simulink model "DAB_IBDC_CONST"  (R2019b)
settings: Solver=ode23t  StartTime=0.0  StopTime=10.0  RelTol=1e-3
libraries: powerlib x18
settings Model: Creator=khduh  LastModifiedBy=khduh

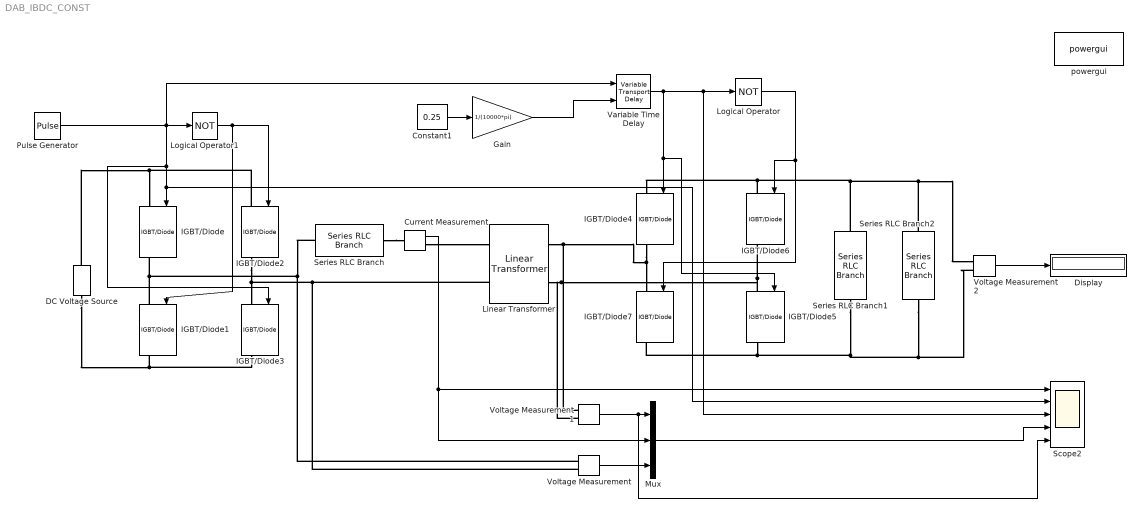
== system DAB_IBDC_CONST ==
  Constant1 : Constant  Value=0.25
  Current Measurement : powerlib/Measurements/Current Measurement  PhasorSimulation=off  OutputType=Complex  PSBequivalent=0
      settings: SourceProductName=Simscape Electrical
  DC Voltage Source : powerlib/Electrical Sources/DC Voltage Source  Amplitude=1000  Measurements=None
      settings: SourceProductName=Simscape Electrical
  Display : Display
  Gain : Gain  Gain=1/(10000*pi)
  IGBT/Diode{,1..7} (8 alike) : powerlib/Power Electronics/IGBT//Diode  Ron=1e-3  Rs=1e5  Cs=inf  Measurements=on
      settings: SourceProductName=Simscape Electrical
  Linear Transformer : powerlib/Elements/Linear Transformer  UNITS=SI  NominalPower=[ 250e6 10000*pi ]  winding1=[500 0 0]  winding2=[250 0 0]  ThreeWindings=off  winding3=[3.15e+05 0.7938 0.084225]  RmLm=[1.0805e+06 2866]  Measurements=None  DataType=on
      settings: SourceProductName=Simscape Electrical
  Logical Operator : Logic  Operator=NOT  AllPortsSameDT=off  OutDataTypeStr=boolean
  Logical Operator1 : Logic  Operator=NOT  AllPortsSameDT=off  OutDataTypeStr=boolean
  Mux : Mux  Inputs=3
  Pulse Generator : DiscretePulseGenerator  PulseType=Time based  Period=1/(10000*pi)  PulseWidth=50
  Scope2 : Scope  NumInputPorts=5
  Series RLC Branch : powerlib/Elements/Series RLC Branch  LConnTagsString=__new0  RConnTagsString=__new0  BranchType=L  Resistance=1  Inductance=.0102e-3  SetiL0=off  InitialCurrent=0  Capacitance=1e-6  Setx0=off  InitialVoltage=0  Measurements=None
      settings: SourceProductName=Simscape Electrical
  Series RLC Branch1 : powerlib/Elements/Series RLC Branch  LConnTagsString=__new0  RConnTagsString=__new0  BranchType=C  Resistance=1  Inductance=.0102e-3  SetiL0=off  InitialCurrent=0  Capacitance=660e-6  Setx0=off  InitialVoltage=0  Measurements=None
      settings: SourceProductName=Simscape Electrical
  Series RLC Branch2 : powerlib/Elements/Series RLC Branch  LConnTagsString=__new0  RConnTagsString=__new0  BranchType=R  Resistance=1  Inductance=.0102e-3  SetiL0=off  InitialCurrent=0  Capacitance=1e-6  Setx0=off  InitialVoltage=0  Measurements=None
      settings: SourceProductName=Simscape Electrical
  Variable Time Delay : VariableTransportDelay  MaximumDelay=10
  Voltage Measurement : powerlib/Measurements/Voltage Measurement  PhasorSimulation=off  OutputType=Complex  PSBequivalent=0
      settings: SourceProductName=Simscape Electrical
  Voltage Measurement1 : powerlib/Measurements/Voltage Measurement  PhasorSimulation=off  OutputType=Complex  PSBequivalent=0
      settings: SourceProductName=Simscape Electrical
  Voltage Measurement2 : powerlib/Measurements/Voltage Measurement  PhasorSimulation=off  OutputType=Complex  PSBequivalent=0
      settings: SourceProductName=Simscape Electrical
  powergui : powerlib/powergui  Priority=1  SimulationMode=Discrete  SampleTime=1e-7  frequency=60  Iterations=50  frequencyindice=0  Pbase=100e6  ErrMax=1e-4  UnitsV=kV  UnitsW=MW  buscounter=0  FunctionMessages=off  echomessages=off  EnableUseOfTLC=off  CurrentSourceSwitches=off  DisableSnubberDevices=off  DisableRonSwitches=off  DisableVfSwitches=off  DisplayEquations=off  AutomaticDiscreteSolvers=off  SolverType=Tustin/Backward Euler (TBE)  Interpol=off  ExternalGateDelay=off  methode=off  Ts=100  x0status=blocks  SPID=on  SwTol=0  HookPort=off  NonlinearTolerance=1e-4  nMaxIteration=100  ContinueOnMaxIteration=off  RestoreLinks=warning  ResistiveCurrentMeasurement=off  Frange=[0:2:500]  Ylog=off  Xlog=on  ShowGrid=off  save=off  variable=ZData  structure=0  ZoomFFT=off  StartTime=0.0  cycles=1  DisplayStyle=1  fundamental=60  FreqAxis=off  MaxFrequency=1000  frequencyindicesteady=1  RmsSteady=1  display=off
      settings: SourceProductName=Simscape Electrical
  wires:
  Voltage Measurement/1 -> Mux/3
  Voltage Measurement1/1 -> Scope2/5, Mux/1
  Mux/1 -> Scope2/4
  Voltage Measurement2/1 -> Display/1
  Gain/1 -> Variable Time Delay/2
  Variable Time Delay/1 -> IGBT/Diode5/1, IGBT/Diode4/1, Scope2/3, Logical Operator/1
  Logical Operator1/1 -> IGBT/Diode2/1, IGBT/Diode1/1
  Constant1/1 -> Gain/1
  Logical Operator/1 -> IGBT/Diode7/1, IGBT/Diode6/1
  Current Measurement/1 -> Mux/2, Scope2/1
  Pulse Generator/1 -> Scope2/2, IGBT/Diode/1, IGBT/Diode3/1, Variable Time Delay/1, Logical Operator1/1
  connections:
  DC Voltage Source/LConn1 -- IGBT/Diode3/RConn1 -- IGBT/Diode1/RConn1
  IGBT/Diode1/LConn1 -- Series RLC Branch/LConn1 -- Voltage Measurement/LConn1 -- IGBT/Diode/RConn1
  IGBT/Diode2/RConn1 -- Voltage Measurement/LConn2 -- Linear Transformer/LConn2 -- IGBT/Diode3/LConn1
  DC Voltage Source/RConn1 -- IGBT/Diode/LConn1 -- IGBT/Diode2/LConn1
  Series RLC Branch/RConn1 -- Current Measurement/LConn1
  Current Measurement/RConn1 -- Linear Transformer/LConn1
  IGBT/Diode6/LConn1 -- Series RLC Branch2/RConn1 -- Voltage Measurement2/LConn1 -- Series RLC Branch1/RConn1 -- IGBT/Diode4/LConn1
  IGBT/Diode4/RConn1 -- Voltage Measurement1/LConn1 -- Linear Transformer/RConn1 -- IGBT/Diode7/LConn1
  IGBT/Diode5/LConn1 -- Voltage Measurement1/LConn2 -- Linear Transformer/RConn2 -- IGBT/Diode6/RConn1
  IGBT/Diode5/RConn1 -- Voltage Measurement2/LConn2 -- Series RLC Branch2/LConn1 -- Series RLC Branch1/LConn1 -- IGBT/Diode7/RConn1
